simulink subsystem "adaptive_sliding"  (R2023b)
settings: Solver=VariableStepAuto  StartTime=0.0  StopTime=10.0  RelTol=1e-3
libraries: simulink_extras x1
settings Model: Creator=Admin  LastModifiedBy=Admin

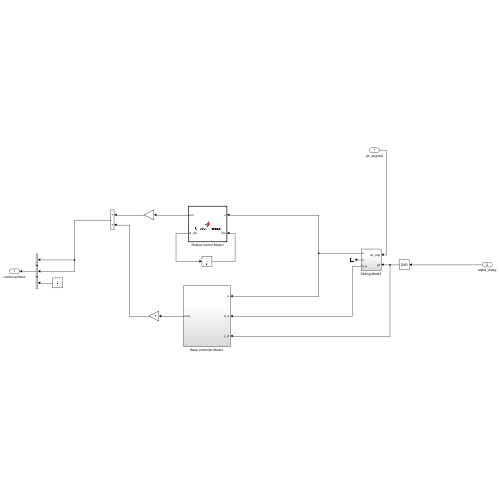
[thumbnail: Simulink's stored preview of the top-level diagram]
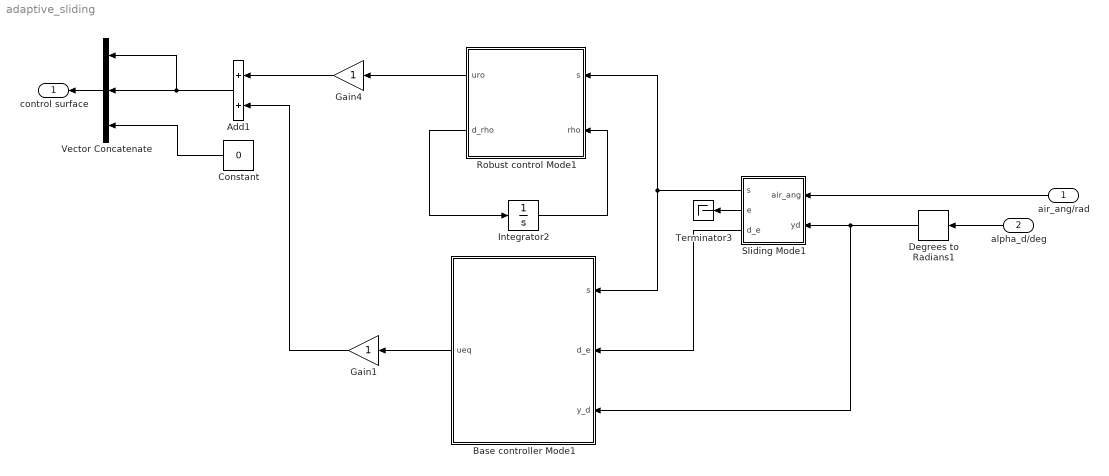
== system adaptive_sliding ==
  air_ang/rad : Inport
  alpha_d/deg : Inport  Port=2
  Add1 : Sum
  Base controller Mode1 : Subsystem
  Constant : Constant  Value=0
  Degrees to Radians1 : simulink_extras/Transformations/Degrees to Radians
  Gain1 : Gain
  Gain4 : Gain
  Integrator2 : Integrator
  Robust control Mode1 : MATLAB Function  TreatAsAtomicUnit=on
  Sliding Mode1 : Subsystem
  Terminator3 : Terminator
  Vector Concatenate : Concatenate  NumInputs=3
  control surface : Outport
  wires:
  Integrator2/1 -> Robust control Mode1/2(rho)
  Sliding Mode1/1(s) -> Base controller Mode1/1(s), Robust control Mode1/1(s)
  Sliding Mode1/3(d_e) -> Base controller Mode1/2(d_e)
  Degrees to Radians1/1 -> Sliding Mode1/2(yd), Base controller Mode1/3(y_d)
  Gain1/1 -> Add1/2
  Robust control Mode1/2(d_rho) -> Integrator2/1
  Sliding Mode1/2(e) -> Terminator3/1
  Gain4/1 -> Add1/1
  Base controller Mode1/1(ueq) -> Gain1/1
  Robust control Mode1/1(uro) -> Gain4/1
  air_ang/rad/1 -> Sliding Mode1/1(air_ang)
  alpha_d/deg/1 -> Degrees to Radians1/1
  Vector Concatenate/1 -> control surface/1
  Add1/1 -> Vector Concatenate/2, Vector Concatenate/1
  Constant/1 -> Vector Concatenate/3

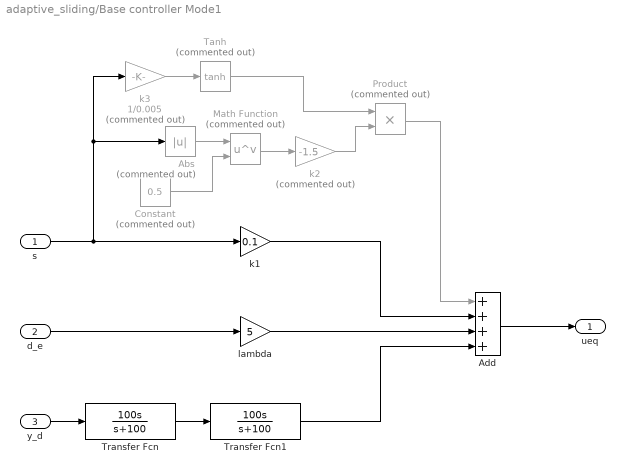
== system adaptive_sliding/Base controller Mode1 ==
  s : Inport
  d_e : Inport  Port=2
  y_d : Inport  Port=3
  Abs : Abs  Commented=on  ZeroCross=off  SaturateOnIntegerOverflow=off
  Add : Sum  Inputs=++++
  Constant : Constant  Commented=on  Value=0.5
  Math Function : Math  Commented=on  Operator=pow
  Product : Product  Commented=on
  Tanh : Trigonometry  Commented=on  Operator=tanh
  Transfer Fcn : TransferFcn  Numerator=[100 0]  Denominator=[1 100]
  Transfer Fcn1 : TransferFcn  Numerator=[100 0]  Denominator=[1 100]
  k1 : Gain  Gain=0.1
  k2 : Gain  Commented=on  Gain=-1.5
  k3 : Gain  Commented=on  Gain=1/0.005
  lambda : Gain  Gain=5
  ueq : Outport
  wires:
  k3/1 -> Tanh/1
  Tanh/1 -> Product/1
  Product/1 -> Add/1
  k2/1 -> Product/2
  Math Function/1 -> k2/1
  Constant/1 -> Math Function/2
  Abs/1 -> Math Function/1
  Transfer Fcn/1 -> Transfer Fcn1/1
  Add/1 -> ueq/1
  d_e/1 -> lambda/1
  y_d/1 -> Transfer Fcn/1
  s/1 -> k1/1, Abs/1, k3/1
  Transfer Fcn1/1 -> Add/4
  lambda/1 -> Add/3
  k1/1 -> Add/2

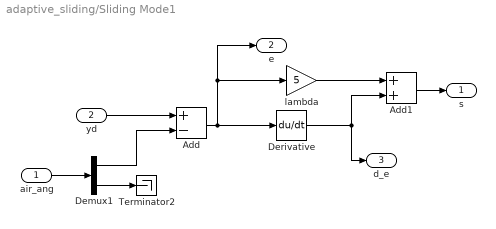
== system adaptive_sliding/Sliding Mode1 ==
  air_ang : Inport
  yd : Inport  Port=2
  Add : Sum  Inputs=+-
  Add1 : Sum
  Demux1 : Demux  Outputs=2
  Derivative : Derivative
  Terminator2 : Terminator
  lambda : Gain  Gain=5
  s : Outport
  e : Outport  Port=2
  d_e : Outport  Port=3
  wires:
  Add1/1 -> s/1
  Derivative/1 -> Add1/2, d_e/1
  lambda/1 -> Add1/1
  Add/1 -> Derivative/1, e/1, lambda/1
  air_ang/1 -> Demux1/1
  Demux1/1 -> Add/2
  yd/1 -> Add/1
  Demux1/2 -> Terminator2/1

== matlab function adaptive_sliding/Robust control Mode1 ==
  data: s input; uro output; rho input; d_rho output
function [uro, d_rho] = S_robust_control(s, rho)
     [d_rho, uro] = robust_control(s, rho);
end
